simulink model "welding_head_three_simulink"  (R2024b)
settings: Solver=ode45  StartTime=0.0  StopTime=8  RelTol=1e-3
libraries: simulink x2
settings Model: Creator=24839  LastModifiedBy=24839

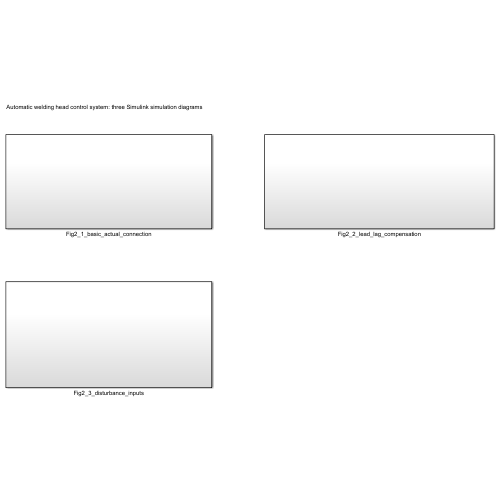
[thumbnail: Simulink's stored preview of the top-level diagram]
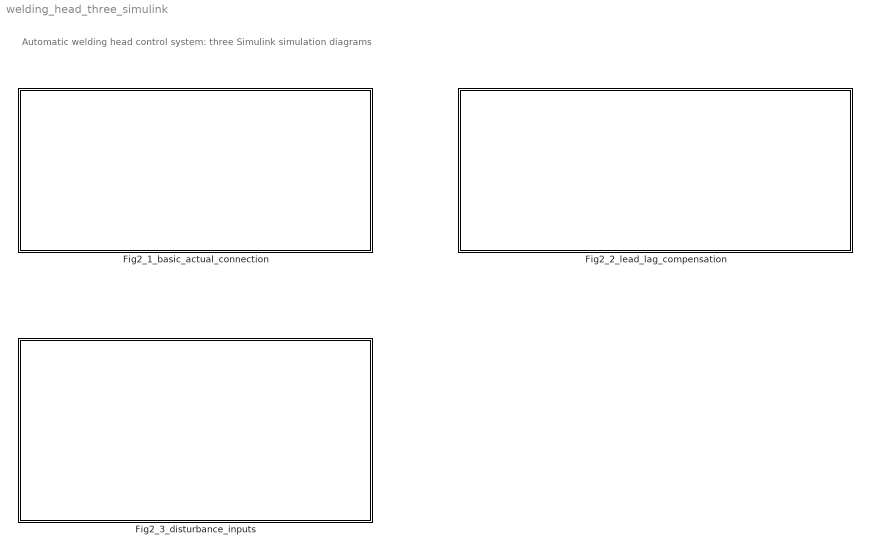
== system welding_head_three_simulink ==
  note: Automatic welding head control system: three Simulink simulation diagrams
  Fig2_1_basic_actual_connection : Subsystem
  Fig2_2_lead_lag_compensation : Subsystem
  Fig2_3_disturbance_inputs : Subsystem

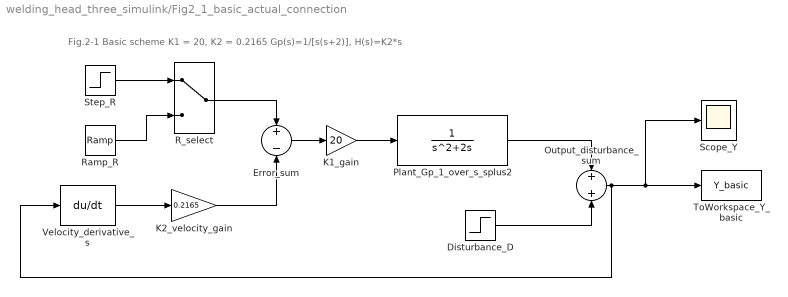
== system welding_head_three_simulink/Fig2_1_basic_actual_connection ==
  note: Fig.2-1 Basic scheme\nK1 = 20, K2 = 0.2165\nGp(s)=1/[s(s+2)], H(s)=K2*s
  Disturbance_D : Step  Time=100  After=0  SampleTime=0
  Error_sum : Sum  Inputs=+-
  K1_gain : Gain  Gain=20
  K2_velocity_gain : Gain  Gain=0.2165
  Output_disturbance_sum : Sum
  Plant_Gp_1_over_s_splus2 : TransferFcn  Denominator=[1 2 0]
  R_select : ManualSwitch
  Ramp_R : simulink/Sources/Ramp  slope=1  start=0  InitialOutput=0
  Scope_Y : Scope
  Step_R : Step  Time=0  SampleTime=0
  ToWorkspace_Y_basic : ToWorkspace  VariableName=Y_basic  SaveFormat=Structure With Time  SampleTime=-1
  Velocity_derivative_s : Derivative
  wires:
  Plant_Gp_1_over_s_splus2/1 -> Output_disturbance_sum/1
  Step_R/1 -> R_select/1
  Ramp_R/1 -> R_select/2
  K2_velocity_gain/1 -> Error_sum/2
  Velocity_derivative_s/1 -> K2_velocity_gain/1
  Error_sum/1 -> K1_gain/1
  R_select/1 -> Error_sum/1
  K1_gain/1 -> Plant_Gp_1_over_s_splus2/1
  Output_disturbance_sum/1 -> Scope_Y/1, ToWorkspace_Y_basic/1, Velocity_derivative_s/1
  Disturbance_D/1 -> Output_disturbance_sum/2

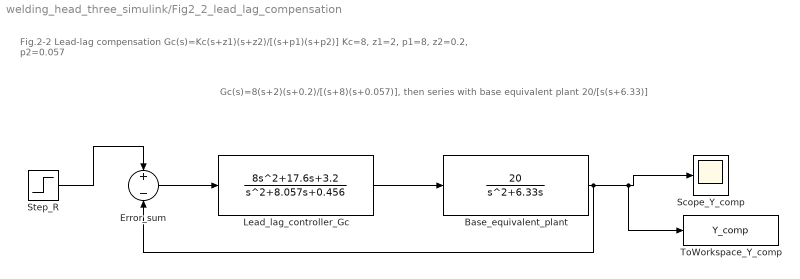
== system welding_head_three_simulink/Fig2_2_lead_lag_compensation ==
  note: Fig.2-2 Lead-lag compensation\nGc(s)=Kc(s+z1)(s+z2)/[(s+p1)(s+p2)]\nKc=8, z1=2, p1=8, z2=0.2, p2=0.057
  note: Gc(s)=8(s+2)(s+0.2)/[(s+8)(s+0.057)], then series with base equivalent plant 20/[s(s+6.33)]
  Base_equivalent_plant : TransferFcn  Numerator=20  Denominator=[1 6.33 0]
  Error_sum : Sum  Inputs=+-
  Lead_lag_controller_Gc : TransferFcn  Numerator=[8 17.6 3.2]  Denominator=[1 8.057 0.456]
  Scope_Y_comp : Scope
  Step_R : Step  Time=0  SampleTime=0
  ToWorkspace_Y_comp : ToWorkspace  VariableName=Y_comp  SaveFormat=Structure With Time  SampleTime=-1
  wires:
  Step_R/1 -> Error_sum/1
  Error_sum/1 -> Lead_lag_controller_Gc/1
  Lead_lag_controller_Gc/1 -> Base_equivalent_plant/1
  Base_equivalent_plant/1 -> Scope_Y_comp/1, ToWorkspace_Y_comp/1, Error_sum/2

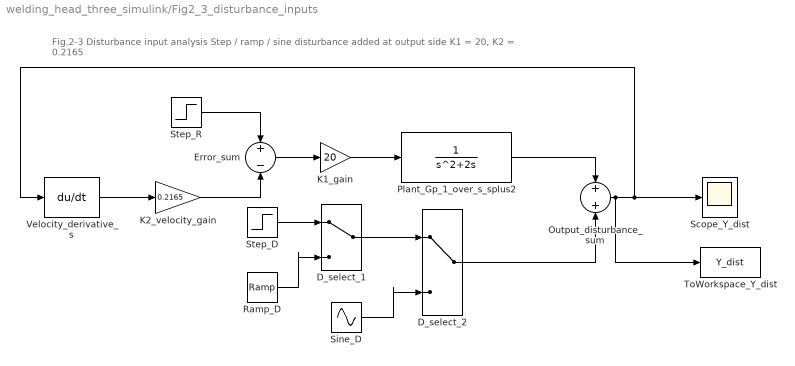
== system welding_head_three_simulink/Fig2_3_disturbance_inputs ==
  note: Fig.2-3 Disturbance input analysis\nStep / ramp / sine disturbance added at output side\nK1 = 20, K2 = 0.2165
  D_select_1 : ManualSwitch
  D_select_2 : ManualSwitch
  Error_sum : Sum  Inputs=+-
  K1_gain : Gain  Gain=20
  K2_velocity_gain : Gain  Gain=0.2165
  Output_disturbance_sum : Sum
  Plant_Gp_1_over_s_splus2 : TransferFcn  Denominator=[1 2 0]
  Ramp_D : simulink/Sources/Ramp  slope=1  start=1  InitialOutput=0
  Scope_Y_dist : Scope
  Sine_D : Sin  Frequency=3  SampleTime=0
  Step_D : Step  SampleTime=0
  Step_R : Step  Time=0  SampleTime=0
  ToWorkspace_Y_dist : ToWorkspace  VariableName=Y_dist  SaveFormat=Structure With Time  SampleTime=-1
  Velocity_derivative_s : Derivative
  wires:
  K2_velocity_gain/1 -> Error_sum/2
  Velocity_derivative_s/1 -> K2_velocity_gain/1
  K1_gain/1 -> Plant_Gp_1_over_s_splus2/1
  Error_sum/1 -> K1_gain/1
  Step_D/1 -> D_select_1/1
  Step_R/1 -> Error_sum/1
  D_select_1/1 -> D_select_2/1
  Ramp_D/1 -> D_select_1/2
  Sine_D/1 -> D_select_2/2
  Plant_Gp_1_over_s_splus2/1 -> Output_disturbance_sum/1
  D_select_2/1 -> Output_disturbance_sum/2
  Output_disturbance_sum/1 -> Velocity_derivative_s/1, Scope_Y_dist/1, ToWorkspace_Y_dist/1
